simulink model "networked"  (R2017b)
settings: Solver=ode45  StartTime=0.0  StopTime=10  RelTol=1e-3  EnableMultiTasking=on
libraries: truetime x5
settings Model: Creator=anton  LastModifiedBy=carlosxavierroserochandi
settings DataIOCC: LimitDataPoints=on  SaveFormat=Array
settings OptimizationCC: ExpressionDepthLimit=2147483647  LifeSpan=inf
settings DebuggingCC: UnderspecifiedInitializationDetection=Classic  MergeDetectMultiDrivingBlocksExec=none  FcnCallInpInsideContextMsg=warning  StateNameClashWarn=warning  SFUnexpectedBacktrackingDiag=warning  SFNoUnconditionalDefaultTransitionDiag=warning  SFExecutionAtInitializationDiag=none
settings HardwareCC: ProdBitPerPointer=32  ProdBitPerSizeT=32  ProdBitPerPtrDiffT=32  ProdLargestAtomicFloat=None  ProdIntDivRoundTo=Undefined  ProdEndianess=Unspecified  ProdWordSize=32  ProdHWDeviceType=32-bit Generic
settings ModelReferenceCC: PropagateSignalLabelsOutOfModel=off
settings CodeAppCC: StateflowObjectComments=on
settings GRTTargetCC: TargetLangStandard=C89/C90 (ANSI)  GeneratePreprocessorConditionals=Disable all
settings ConfigComp: CovMetricSettings=dw  CovHtmlReporting=on  CovSaveCumulativeToWorkspaceVar=on  CovSaveSingleToWorkspaceVar=on  CovExternalEMLEnable=off

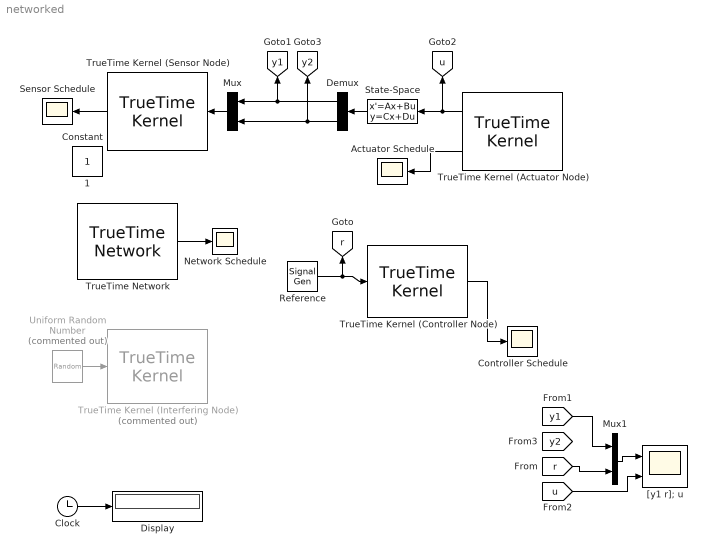
== system networked ==
  Actuator Schedule : Scope
  Clock : Clock
  Controller Schedule : Scope
  Demux : Demux  Outputs=2
  Display : Display
  Mux : Mux  Inputs=2
  Mux1 : Mux  Inputs=2
  Network Schedule : Scope
  Reference : SignalGenerator  WaveForm=square  Amplitude=5  Frequency=0.125
  Sensor Schedule : Scope
  State-Space : StateSpace  A=[0 -23.8095; 0 0];  B=[0; -23.8095];  C=[1 0; 0 1]  D=[0; 0]  InitialCondition=0
  TrueTime Kernel (Actuator Node) : truetime/TrueTime Kernel  sfun=actuator_init  args=[]  ninputsoutputs=[0 1]  ntriggers=0  trigtype=rising  nwnodenbr=4  clockoffsetdrift=[0 0]  schedoutput=on  battery=off  poweroutput=off  label=1: 4
  TrueTime Kernel (Controller Node) : truetime/TrueTime Kernel  sfun=controller_init  args=0.0  ninputsoutputs=[1 0]  ntriggers=0  trigtype=rising  nwnodenbr=3  clockoffsetdrift=[0 0]  schedoutput=on  battery=off  poweroutput=off  label=1: 3
  TrueTime Kernel (Interfering Node) : truetime/TrueTime Kernel  Commented=on  sfun=interference_init  args=0.3  ninputsoutputs=[1 0]  ntriggers=0  trigtype=rising  nwnodenbr=1  clockoffsetdrift=[0 0]  schedoutput=off  battery=off  poweroutput=off  label=1: 1
  TrueTime Kernel (Sensor Node) : truetime/TrueTime Kernel  sfun=sensor_init  args=[]  ninputsoutputs=[2 0]  ntriggers=0  trigtype=rising  nwnodenbr=2  clockoffsetdrift=[0 0]  schedoutput=on  battery=off  poweroutput=off  label=1: 2
  TrueTime Network : truetime/TrueTime Network  nwtype=CSMA/CD (Ethernet)  nwnbr=1  nnodes=4  rate=80000  minsize=80  lossprob=0  seed=0  bandwidths=[0.5 0.25 0.25]  slotsize=80  schedule=[1 2 1 3]  memsize=80000  buftype=Common buffer  overflow=Retransmit  dynSchedule=[]  miniSlotSize=40  NIT=0  QSortMode=FIFO  sync=0  irtSchedule=0  nrtLength=0  nodeGraph=0  scheduleoutput=on
  Uniform Random Number : UniformRandomNumber  Commented=on  Minimum=0  SampleTime=0.001
  "[y1 r]; u" : Scope  NumInputPorts=2
  1 : Constant  IOType=siggen
  Constant : Constant  IOType=siggen
  tag scope: r=global, u=global, y1=global, y2=global
  wires:
  TrueTime Network/1 -> Network Schedule/1
  Mux1/1 -> "[y1 r]; u"/1
  Clock/1 -> Display/1
  Reference/1 -> TrueTime Kernel (Controller Node)/1, [r]
  TrueTime Kernel (Controller Node)/1 -> Controller Schedule/1
  [y1] -> Mux1/1
  [u] -> "[y1 r]; u"/2
  Uniform Random Number/1 -> TrueTime Kernel (Interfering Node)/1
  TrueTime Kernel (Sensor Node)/1 -> Sensor Schedule/1
  TrueTime Kernel (Actuator Node)/1 -> [u], State-Space/1
  TrueTime Kernel (Actuator Node)/2 -> Actuator Schedule/1
  Mux/1 -> TrueTime Kernel (Sensor Node)/1
  [r] -> Mux1/2
  State-Space/1 -> Demux/1
  Demux/1 -> [y1], Mux/1
  Demux/2 -> [y2], Mux/2
